simulink model "AV10_PRIMER1"  (R2018a)
settings: Solver=VariableStepAuto  StartTime=0.0  StopTime=100  RelTol=1e-3
values from neighbouring files (symbols this model uses):
  q0 = -1.1901    [AV10_ZADACHA1.m]    (also in AV9_PRIMER2_VREDNOSTI.m = -62.3782; AV9_PRIMER4.m = 1.9573; AV9_PRIMER5.m = 1.8649; AV_10_PRIMER1.m = 1.512)
  q1 = 0.8945    [AV10_ZADACHA1.m]    (also in AV9_PRIMER2_VREDNOSTI.m = 122.0694; AV9_PRIMER4.m = -1.6594; AV9_PRIMER5.m = -1.8649; AV_10_PRIMER1.m = -1.423)
  q2 = -0.2805    [AV10_ZADACHA1.m]    (also in AV9_PRIMER2_VREDNOSTI.m = -59.9743; AV9_PRIMER4.m = 0.6675; AV9_PRIMER5.m = 0.2403; AV_10_PRIMER1.m = 0.44)
  T = 160    [AV10_ZADACHA1.m]    (also in AV9_PRIMER4.m = 16; AV9_PRIMER5.m = 4; AV_10_PRIMER1.m = 8)
settings Model: Creator=DD  LastModifiedBy=DD

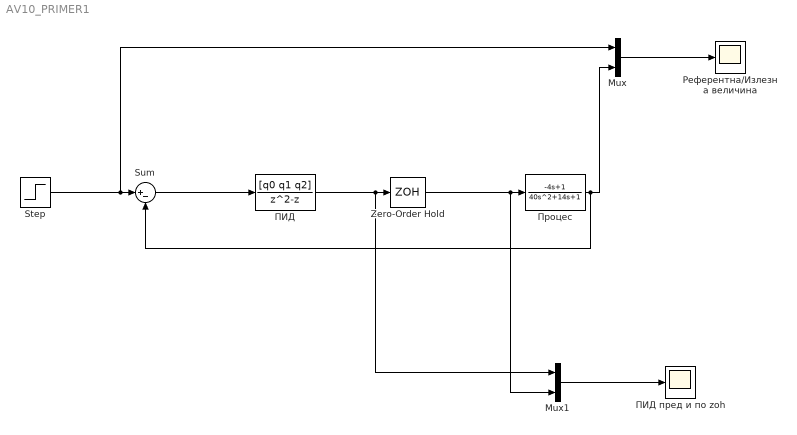
== system AV10_PRIMER1 ==
  Mux : Mux  Inputs=2
  Mux1 : Mux  Inputs=2
  Step : Step  SampleTime=0
  Sum : Sum  Inputs=|+-
  Zero-Order Hold : ZeroOrderHold  SampleTime=-1
  "ПИД " : DiscreteTransferFcn  Numerator=[q0 q1 q2]  Denominator=[1 -1 0]  SampleTime=T
  "ПИД пред и по zoh " : Scope
  "Процес " : TransferFcn  Numerator=[-4 1]  Denominator=[40 14 1]
  Референтна/Излезна величина : Scope
  wires:
  Mux/1 -> Референтна/Излезна величина/1
  Zero-Order Hold/1 -> Mux1/2, "Процес "/1
  "ПИД "/1 -> Mux1/1, Zero-Order Hold/1
  Sum/1 -> "ПИД "/1
  "Процес "/1 -> Sum/2, Mux/2
  Mux1/1 -> "ПИД пред и по zoh "/1
  Step/1 -> Mux/1, Sum/1
